simulink library "thermochemical"  (R2017b)
settings: Solver=VariableStepAuto  StartTime=0.0  StopTime=10.0  RelTol=1e-3
values from neighbouring files (symbols this model uses):
  c = conversion_factors()    [blk_clausius_clapeyron.m]    (also in blk_clausius_clapeyron_no_popup.m; blk_cold_room_closed_dry_air.m; blk_reactor_BaCl2_NH3_no_walls.m; blk_reactor_BaCl2_NH3_no_walls_state_space.m)
  cp = metal.cp    [blk_wall_simple.m]    (also in get_metal_properties.m = 390)
  fluid = get_param(blk,'fluid')    [blk_thermodynamic_properties_nonsaturated.m]    (also in blk_thermodynamic_properties_nonsaturated_interpreted.m; blk_thermodynamic_properties_saturated.m; blk_thermodynamic_properties_saturated_interpreted.m; blk_thermodynamic_properties_saturated_mix.m)
  gas = get_material_properties(x.gasName)    [blk_reactor_BaCl2_NH3_cylindrical_no_walls_fun1.m]
  h = get_param(gcb,'ObjectParameters')    [get_param_eval.m]
  rho = metal.rho    [blk_wall_simple.m]    (also in get_metal_properties.m = 8940)
  s = solve(eq,dx,'ReturnConditions',true)    [LMTD_inv.m]    (also in blk_wall_simple.m = get_param_eval(blk,'s'))
  u_gas_at_T_ref = -R * T_ref    [blk_reactor_BaCl2_NH3_no_walls.m]    (also in blk_reactor_BaCl2_NH3_no_walls_state_space.m)
undefined symbols (not defined in the file or in its folder): b_motor, BaCl2, beta, CoolProp, cP_binder, cP_gas, cP_s0, cv, dh_r_0, ENG, heat_exchanger_epsilonNTU_inv_simulink, heat_exchanger_epsilonNTU_simulink, J_motor, K_cin, kappa, Km_motor, La_motor, lookup2D_BreakPoint2, M_binder, N_binder, N_gas_free_volume_init, N_salt, NH3, nh3_v3, nu, P, phase, PID_D_motor, PID_I_motor, PID_P_motor, Ra_motor, Reactor_phase, T, T1, T2, T_init, Tr_init, Tr_ref, U_binder_at_Tr_ref, U_salt_at_X0_Tr_ref, Ur_init, V_void, Valve_regime, Vmax_motor, w_init_motor, X_init
libraries: thermochemical x247, simulink x54, dspsigops x3
(part 5 of 12)

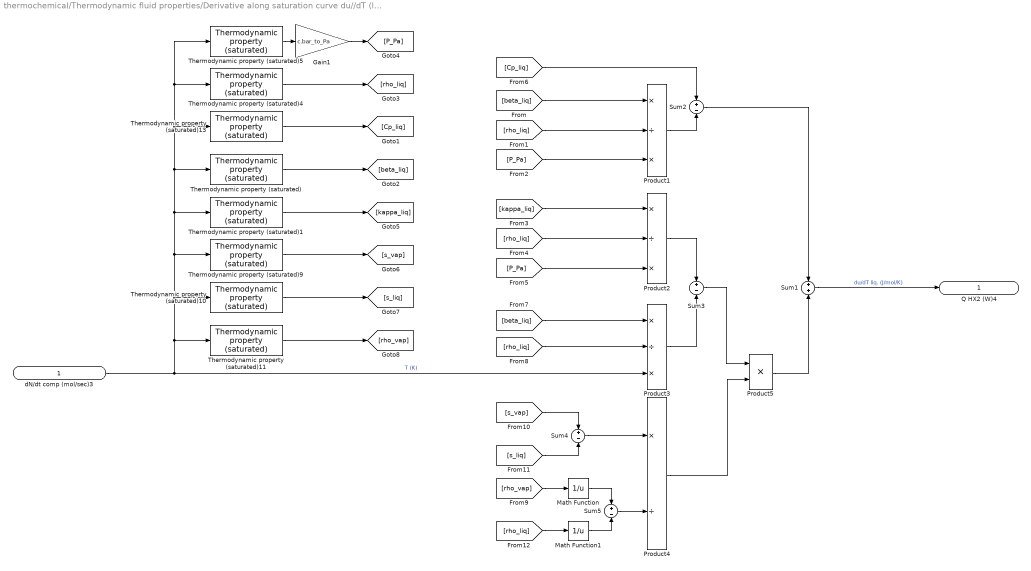
== system thermochemical/Thermodynamic fluid properties/Derivative along saturation curve du//dT (liq.) ==
  dN/dt comp (mol/sec)3 : Inport
  Gain1 : Gain  Gain=c.bar_to_Pa
  Math Function : Math  Operator=reciprocal  SaturateOnIntegerOverflow=on
  Math Function1 : Math  Operator=reciprocal  SaturateOnIntegerOverflow=on
  Product1 : Product  Inputs=*/*
  Product2 : Product  Inputs=*/*
  Product3 : Product  Inputs=*/*
  Product4 : Product  Inputs=*/
  Product5 : Product  Inputs=**
  Sum1 : Sum
  Sum{2..5} (4 alike) : Sum  Inputs=+-
  Thermodynamic property (saturated) : thermochemical/Thermodynamic fluid properties/Thermodynamic  property (saturated)  sel=beta(T) liq. (1/K)  fluid=fluid  lookup1D_BreakPoint1=fluid.sat.T  lookup1D_Data=fluid.sat.liq.beta
      settings: SourceProductName=@ Thermochemical
  Thermodynamic property (saturated)1 : thermochemical/Thermodynamic fluid properties/Thermodynamic  property (saturated)  sel=kappa(T) liq. (1/Pa)  fluid=fluid  lookup1D_BreakPoint1=fluid.sat.T  lookup1D_Data=fluid.sat.liq.kappa
      settings: SourceProductName=@ Thermochemical
  Thermodynamic property (saturated)10 : thermochemical/Thermodynamic fluid properties/Thermodynamic  property (saturated)  sel=s(T) liq. (J/K/mol)  fluid=fluid  lookup1D_BreakPoint1=fluid.sat.T  lookup1D_Data=fluid.sat.liq.s_molar
      settings: SourceProductName=@ Thermochemical
  Thermodynamic property (saturated)11 : thermochemical/Thermodynamic fluid properties/Thermodynamic  property (saturated)  sel=rho(T) vap. (mol/m3)  fluid=fluid  lookup1D_BreakPoint1=fluid.sat.T  lookup1D_Data=fluid.sat.vap.rho_molar
      settings: SourceProductName=@ Thermochemical
  Thermodynamic property (saturated)13 : thermochemical/Thermodynamic fluid properties/Thermodynamic  property (saturated)  sel=Cp(T) liq. (J/K/mol)  fluid=fluid  lookup1D_BreakPoint1=fluid.sat.T  lookup1D_Data=fluid.sat.liq.Cp_molar
      settings: SourceProductName=@ Thermochemical
  Thermodynamic property (saturated)4 : thermochemical/Thermodynamic fluid properties/Thermodynamic  property (saturated)  sel=rho(T) liq. (mol/m3)  fluid=fluid  lookup1D_BreakPoint1=fluid.sat.T  lookup1D_Data=fluid.sat.liq.rho_molar
      settings: SourceProductName=@ Thermochemical
  Thermodynamic property (saturated)5 : thermochemical/Thermodynamic fluid properties/Thermodynamic  property (saturated)  sel=P(T) (bar)  fluid=nh3_v4  lookup1D_BreakPoint1=nh3_v4.sat.T  lookup1D_Data=nh3_v4.sat.Psat
      settings: SourceProductName=@ Thermochemical
  Thermodynamic property (saturated)9 : thermochemical/Thermodynamic fluid properties/Thermodynamic  property (saturated)  sel=s(T) vap. (J/K/mol)  fluid=fluid  lookup1D_BreakPoint1=fluid.sat.T  lookup1D_Data=fluid.sat.vap.s_molar
      settings: SourceProductName=@ Thermochemical
  Q HX2 (W)4 : Outport
  wires:
  Thermodynamic property (saturated)11/1 -> [rho_vap]
  Thermodynamic property (saturated)10/1 -> [s_liq]
  Thermodynamic property (saturated)9/1 -> [s_vap]
  Thermodynamic property (saturated)1/1 -> [kappa_liq]
  Gain1/1 -> [P_Pa]
  Thermodynamic property (saturated)5/1 -> Gain1/1
  Thermodynamic property (saturated)4/1 -> [rho_liq]
  Thermodynamic property (saturated)/1 -> [beta_liq]
  Thermodynamic property (saturated)13/1 -> [Cp_liq]
  Sum1/1 -> Q HX2 (W)4/1  "du/dT liq. (J/mol/K)"
  [Cp_liq] -> Sum2/1
  Product1/1 -> Sum2/2
  [beta_liq] -> Product1/1
  [rho_liq] -> Product1/2
  Sum2/1 -> Sum1/1
  [P_Pa] -> Product1/3
  dN/dt comp (mol/sec)3/1 -> Product3/3, Thermodynamic property (saturated)5/1, Thermodynamic property (saturated)4/1, Thermodynamic property (saturated)13/1, Thermodynamic property (saturated)/1, Thermodynamic property (saturated)1/1, Thermodynamic property (saturated)9/1, Thermodynamic property (saturated)10/1, Thermodynamic property (saturated)11/1  "T (K)"
  [kappa_liq] -> Product2/1
  [rho_liq] -> Product2/2
  [P_Pa] -> Product2/3
  Product2/1 -> Sum3/1
  [rho_liq] -> Product3/2
  [beta_liq] -> Product3/1
  Product3/1 -> Sum3/2
  [s_vap] -> Sum4/1
  [s_liq] -> Sum4/2
  Sum4/1 -> Product4/1
  Sum5/1 -> Product4/2
  [rho_liq] -> Math Function1/1
  [rho_vap] -> Math Function/1
  Math Function/1 -> Sum5/1
  Math Function1/1 -> Sum5/2
  Sum3/1 -> Product5/1
  Product4/1 -> Product5/2
  Product5/1 -> Sum1/2

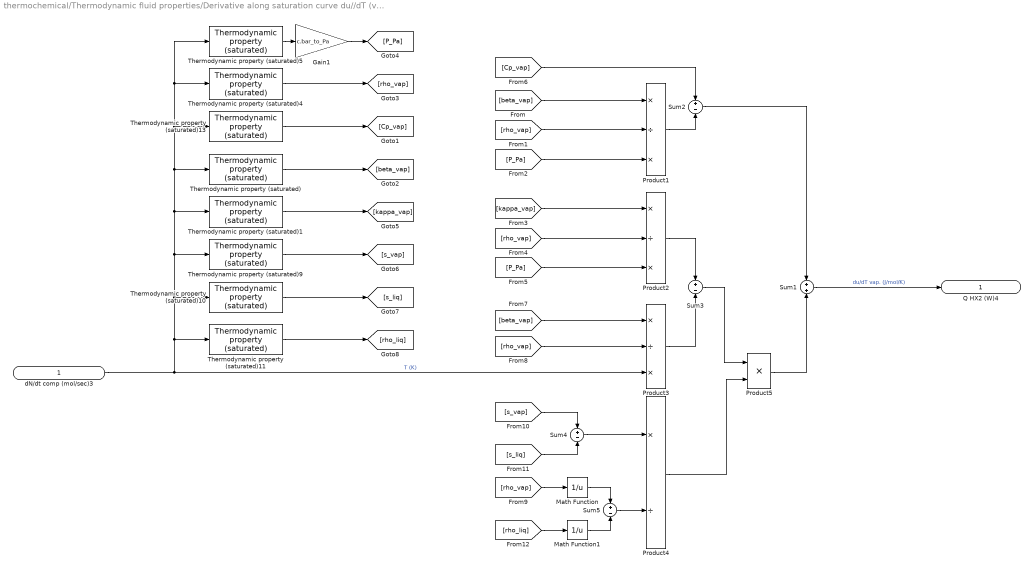
== system thermochemical/Thermodynamic fluid properties/Derivative along saturation curve du//dT (vap.) ==
  dN/dt comp (mol/sec)3 : Inport
  Gain1 : Gain  Gain=c.bar_to_Pa
  Math Function : Math  Operator=reciprocal  SaturateOnIntegerOverflow=on
  Math Function1 : Math  Operator=reciprocal  SaturateOnIntegerOverflow=on
  Product1 : Product  Inputs=*/*
  Product2 : Product  Inputs=*/*
  Product3 : Product  Inputs=*/*
  Product4 : Product  Inputs=*/
  Product5 : Product  Inputs=**
  Sum1 : Sum
  Sum{2..5} (4 alike) : Sum  Inputs=+-
  Thermodynamic property (saturated) : thermochemical/Thermodynamic fluid properties/Thermodynamic  property (saturated)  sel=beta(T) vap. (1/K)  fluid=fluid  lookup1D_BreakPoint1=fluid.sat.T  lookup1D_Data=fluid.sat.vap.beta
      settings: SourceProductName=@ Thermochemical
  Thermodynamic property (saturated)1 : thermochemical/Thermodynamic fluid properties/Thermodynamic  property (saturated)  sel=kappa(T) vap. (1/Pa)  fluid=fluid  lookup1D_BreakPoint1=fluid.sat.T  lookup1D_Data=fluid.sat.vap.kappa
      settings: SourceProductName=@ Thermochemical
  Thermodynamic property (saturated)10 : thermochemical/Thermodynamic fluid properties/Thermodynamic  property (saturated)  sel=s(T) liq. (J/K/mol)  fluid=fluid  lookup1D_BreakPoint1=fluid.sat.T  lookup1D_Data=fluid.sat.liq.s_molar
      settings: SourceProductName=@ Thermochemical
  Thermodynamic property (saturated)11 : thermochemical/Thermodynamic fluid properties/Thermodynamic  property (saturated)  sel=rho(T) liq. (mol/m3)  fluid=fluid  lookup1D_BreakPoint1=fluid.sat.T  lookup1D_Data=fluid.sat.liq.rho_molar
      settings: SourceProductName=@ Thermochemical
  Thermodynamic property (saturated)13 : thermochemical/Thermodynamic fluid properties/Thermodynamic  property (saturated)  sel=Cp(T) vap. (J/K/mol)  fluid=fluid  lookup1D_BreakPoint1=fluid.sat.T  lookup1D_Data=fluid.sat.vap.Cp_molar
      settings: SourceProductName=@ Thermochemical
  Thermodynamic property (saturated)4 : thermochemical/Thermodynamic fluid properties/Thermodynamic  property (saturated)  sel=rho(T) vap. (mol/m3)  fluid=fluid  lookup1D_BreakPoint1=fluid.sat.T  lookup1D_Data=fluid.sat.vap.rho_molar
      settings: SourceProductName=@ Thermochemical
  Thermodynamic property (saturated)5 : thermochemical/Thermodynamic fluid properties/Thermodynamic  property (saturated)  sel=P(T) (bar)  fluid=nh3_v4  lookup1D_BreakPoint1=nh3_v4.sat.T  lookup1D_Data=nh3_v4.sat.Psat
      settings: SourceProductName=@ Thermochemical
  Thermodynamic property (saturated)9 : thermochemical/Thermodynamic fluid properties/Thermodynamic  property (saturated)  sel=s(T) vap. (J/K/mol)  fluid=fluid  lookup1D_BreakPoint1=fluid.sat.T  lookup1D_Data=fluid.sat.vap.s_molar
      settings: SourceProductName=@ Thermochemical
  Q HX2 (W)4 : Outport
  wires:
  Product5/1 -> Sum1/2
  Product4/1 -> Product5/2
  Sum3/1 -> Product5/1
  Math Function1/1 -> Sum5/2
  Math Function/1 -> Sum5/1
  [rho_vap] -> Math Function/1
  [rho_liq] -> Math Function1/1
  Sum5/1 -> Product4/2
  Sum4/1 -> Product4/1
  [s_liq] -> Sum4/2
  [s_vap] -> Sum4/1
  Product3/1 -> Sum3/2
  [beta_vap] -> Product3/1
  [rho_vap] -> Product3/2
  Product2/1 -> Sum3/1
  [P_Pa] -> Product2/3
  [rho_vap] -> Product2/2
  [kappa_vap] -> Product2/1
  dN/dt comp (mol/sec)3/1 -> Thermodynamic property (saturated)11/1, Thermodynamic property (saturated)10/1, Thermodynamic property (saturated)9/1, Thermodynamic property (saturated)1/1, Thermodynamic property (saturated)/1, Thermodynamic property (saturated)13/1, Thermodynamic property (saturated)4/1, Thermodynamic property (saturated)5/1, Product3/3  "T (K)"
  [P_Pa] -> Product1/3
  Sum2/1 -> Sum1/1
  [rho_vap] -> Product1/2
  [beta_vap] -> Product1/1
  Product1/1 -> Sum2/2
  [Cp_vap] -> Sum2/1
  Sum1/1 -> Q HX2 (W)4/1  "du/dT vap. (J/mol/K)"
  Thermodynamic property (saturated)13/1 -> [Cp_vap]
  Thermodynamic property (saturated)/1 -> [beta_vap]
  Thermodynamic property (saturated)4/1 -> [rho_vap]
  Thermodynamic property (saturated)5/1 -> Gain1/1
  Gain1/1 -> [P_Pa]
  Thermodynamic property (saturated)1/1 -> [kappa_vap]
  Thermodynamic property (saturated)9/1 -> [s_vap]
  Thermodynamic property (saturated)10/1 -> [s_liq]
  Thermodynamic property (saturated)11/1 -> [rho_liq]

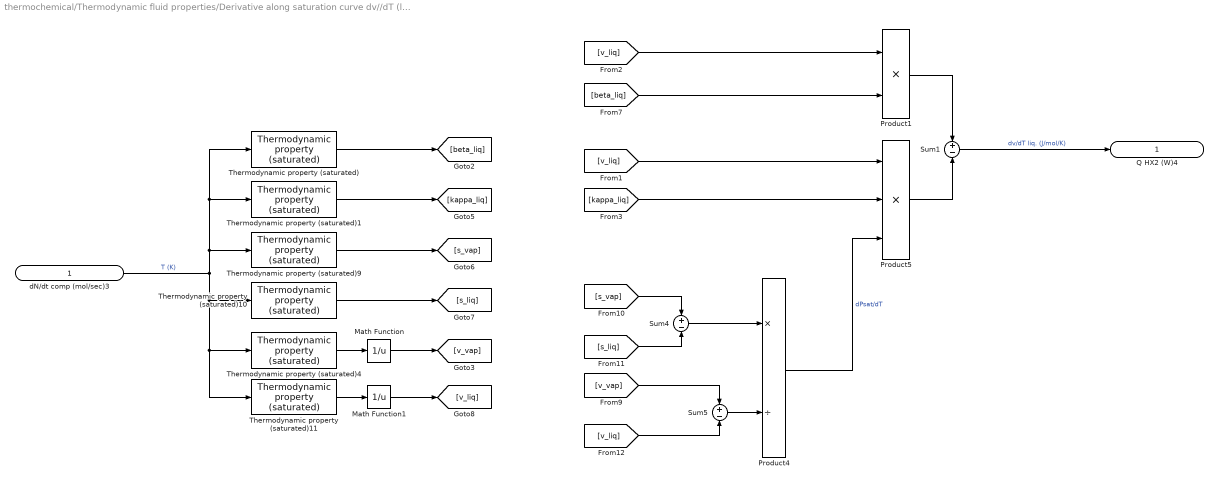
== system thermochemical/Thermodynamic fluid properties/Derivative along saturation curve dv//dT (liq.) ==
  dN/dt comp (mol/sec)3 : Inport
  Math Function : Math  Operator=reciprocal  SaturateOnIntegerOverflow=on
  Math Function1 : Math  Operator=reciprocal  SaturateOnIntegerOverflow=on
  Product1 : Product  Inputs=**
  Product4 : Product  Inputs=*/
  Product5 : Product  Inputs=***
  Sum1 : Sum  Inputs=+-
  Sum4 : Sum  Inputs=+-
  Sum5 : Sum  Inputs=+-
  Thermodynamic property (saturated) : thermochemical/Thermodynamic fluid properties/Thermodynamic  property (saturated)  sel=beta(T) liq. (1/K)  fluid=fluid  lookup1D_BreakPoint1=fluid.sat.T  lookup1D_Data=fluid.sat.liq.beta
      settings: SourceProductName=@ Thermochemical
  Thermodynamic property (saturated)1 : thermochemical/Thermodynamic fluid properties/Thermodynamic  property (saturated)  sel=kappa(T) liq. (1/Pa)  fluid=fluid  lookup1D_BreakPoint1=fluid.sat.T  lookup1D_Data=fluid.sat.liq.kappa
      settings: SourceProductName=@ Thermochemical
  Thermodynamic property (saturated)10 : thermochemical/Thermodynamic fluid properties/Thermodynamic  property (saturated)  sel=s(T) liq. (J/K/mol)  fluid=fluid  lookup1D_BreakPoint1=fluid.sat.T  lookup1D_Data=fluid.sat.liq.s_molar
      settings: SourceProductName=@ Thermochemical
  Thermodynamic property (saturated)11 : thermochemical/Thermodynamic fluid properties/Thermodynamic  property (saturated)  sel=rho(T) liq. (mol/m3)  fluid=fluid  lookup1D_BreakPoint1=fluid.sat.T  lookup1D_Data=fluid.sat.liq.rho_molar
      settings: SourceProductName=@ Thermochemical
  Thermodynamic property (saturated)4 : thermochemical/Thermodynamic fluid properties/Thermodynamic  property (saturated)  sel=rho(T) vap. (mol/m3)  fluid=fluid  lookup1D_BreakPoint1=fluid.sat.T  lookup1D_Data=fluid.sat.vap.rho_molar
      settings: SourceProductName=@ Thermochemical
  Thermodynamic property (saturated)9 : thermochemical/Thermodynamic fluid properties/Thermodynamic  property (saturated)  sel=s(T) vap. (J/K/mol)  fluid=fluid  lookup1D_BreakPoint1=fluid.sat.T  lookup1D_Data=fluid.sat.vap.s_molar
      settings: SourceProductName=@ Thermochemical
  Q HX2 (W)4 : Outport
  wires:
  Product1/1 -> Sum1/1
  [v_liq] -> Product1/1
  [v_liq] -> Product5/1
  Math Function1/1 -> [v_liq]
  Math Function/1 -> [v_vap]
  Product5/1 -> Sum1/2
  Product4/1 -> Product5/3  "dPsat/dT"
  [v_liq] -> Sum5/2
  [v_vap] -> Sum5/1
  Sum5/1 -> Product4/2
  Sum4/1 -> Product4/1
  [s_liq] -> Sum4/2
  [s_vap] -> Sum4/1
  [beta_liq] -> Product1/2
  [kappa_liq] -> Product5/2
  dN/dt comp (mol/sec)3/1 -> Thermodynamic property (saturated)9/1, Thermodynamic property (saturated)1/1, Thermodynamic property (saturated)/1, Thermodynamic property (saturated)10/1, Thermodynamic property (saturated)4/1, Thermodynamic property (saturated)11/1  "T (K)"
  Sum1/1 -> Q HX2 (W)4/1  "dv/dT liq. (J/mol/K)"
  Thermodynamic property (saturated)/1 -> [beta_liq]
  Thermodynamic property (saturated)4/1 -> Math Function/1
  Thermodynamic property (saturated)1/1 -> [kappa_liq]
  Thermodynamic property (saturated)9/1 -> [s_vap]
  Thermodynamic property (saturated)10/1 -> [s_liq]
  Thermodynamic property (saturated)11/1 -> Math Function1/1

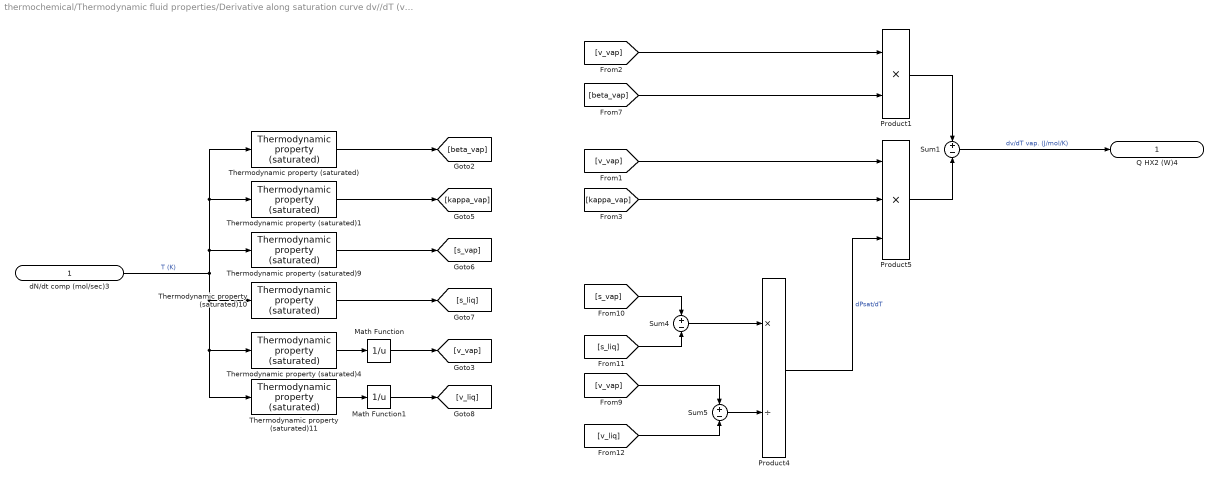
== system thermochemical/Thermodynamic fluid properties/Derivative along saturation curve dv//dT (vap.) ==
  dN/dt comp (mol/sec)3 : Inport
  Math Function : Math  Operator=reciprocal  SaturateOnIntegerOverflow=on
  Math Function1 : Math  Operator=reciprocal  SaturateOnIntegerOverflow=on
  Product1 : Product  Inputs=**
  Product4 : Product  Inputs=*/
  Product5 : Product  Inputs=***
  Sum1 : Sum  Inputs=+-
  Sum4 : Sum  Inputs=+-
  Sum5 : Sum  Inputs=+-
  Thermodynamic property (saturated) : thermochemical/Thermodynamic fluid properties/Thermodynamic  property (saturated)  sel=beta(T) vap. (1/K)  fluid=fluid  lookup1D_BreakPoint1=fluid.sat.T  lookup1D_Data=fluid.sat.vap.beta
      settings: SourceProductName=@ Thermochemical
  Thermodynamic property (saturated)1 : thermochemical/Thermodynamic fluid properties/Thermodynamic  property (saturated)  sel=kappa(T) vap. (1/Pa)  fluid=fluid  lookup1D_BreakPoint1=fluid.sat.T  lookup1D_Data=fluid.sat.vap.kappa
      settings: SourceProductName=@ Thermochemical
  Thermodynamic property (saturated)10 : thermochemical/Thermodynamic fluid properties/Thermodynamic  property (saturated)  sel=s(T) liq. (J/K/mol)  fluid=fluid  lookup1D_BreakPoint1=fluid.sat.T  lookup1D_Data=fluid.sat.liq.s_molar
      settings: SourceProductName=@ Thermochemical
  Thermodynamic property (saturated)11 : thermochemical/Thermodynamic fluid properties/Thermodynamic  property (saturated)  sel=rho(T) liq. (mol/m3)  fluid=fluid  lookup1D_BreakPoint1=fluid.sat.T  lookup1D_Data=fluid.sat.liq.rho_molar
      settings: SourceProductName=@ Thermochemical
  Thermodynamic property (saturated)4 : thermochemical/Thermodynamic fluid properties/Thermodynamic  property (saturated)  sel=rho(T) vap. (mol/m3)  fluid=fluid  lookup1D_BreakPoint1=fluid.sat.T  lookup1D_Data=fluid.sat.vap.rho_molar
      settings: SourceProductName=@ Thermochemical
  Thermodynamic property (saturated)9 : thermochemical/Thermodynamic fluid properties/Thermodynamic  property (saturated)  sel=s(T) vap. (J/K/mol)  fluid=fluid  lookup1D_BreakPoint1=fluid.sat.T  lookup1D_Data=fluid.sat.vap.s_molar
      settings: SourceProductName=@ Thermochemical
  Q HX2 (W)4 : Outport
  wires:
  Thermodynamic property (saturated)11/1 -> Math Function1/1
  Thermodynamic property (saturated)10/1 -> [s_liq]
  Thermodynamic property (saturated)9/1 -> [s_vap]
  Thermodynamic property (saturated)1/1 -> [kappa_vap]
  Thermodynamic property (saturated)4/1 -> Math Function/1
  Thermodynamic property (saturated)/1 -> [beta_vap]
  Sum1/1 -> Q HX2 (W)4/1  "dv/dT vap. (J/mol/K)"
  dN/dt comp (mol/sec)3/1 -> Thermodynamic property (saturated)11/1, Thermodynamic property (saturated)4/1, Thermodynamic property (saturated)10/1, Thermodynamic property (saturated)/1, Thermodynamic property (saturated)1/1, Thermodynamic property (saturated)9/1  "T (K)"
  [kappa_vap] -> Product5/2
  [beta_vap] -> Product1/2
  [s_vap] -> Sum4/1
  [s_liq] -> Sum4/2
  Sum4/1 -> Product4/1
  Sum5/1 -> Product4/2
  [v_vap] -> Sum5/1
  [v_liq] -> Sum5/2
  Product4/1 -> Product5/3  "dPsat/dT"
  Product5/1 -> Sum1/2
  Math Function/1 -> [v_vap]
  Math Function1/1 -> [v_liq]
  [v_vap] -> Product5/1
  [v_vap] -> Product1/1
  Product1/1 -> Sum1/1

== system thermochemical/Thermodynamic fluid properties/Derivative in the two-phase region ∂u//∂T|v ==
  dN/dt comp (mol/sec)1 : Inport
  dN/dt comp (mol/sec)2 : Inport  Port=2
  Derivative along saturation curve du/dT (liq.) : thermochemical/Thermodynamic fluid properties/Derivative along saturation curve du//dT (liq.)  fluid=fluid
      settings: SourceProductName=@ Thermochemical
  Derivative along saturation curve du/dT (vap.) : thermochemical/Thermodynamic fluid properties/Derivative along saturation curve du//dT (vap.)  fluid=fluid
      settings: SourceProductName=@ Thermochemical
  Derivative in the two-phase region ∂χ/∂T|v : thermochemical/Thermodynamic fluid properties/Derivative in the two-phase region ∂χ//∂T|v  fluid=fluid
      settings: SourceProductName=@ Thermochemical
  Product1 : Product  Inputs=**
  Product2 : Product  Inputs=**
  Sum1 : Sum  Inputs=+-
  Sum2 : Sum  Inputs=+-
  Sum3 : Sum  Inputs=+++
  Thermodynamic property (saturated) : thermochemical/Thermodynamic fluid properties/Thermodynamic  property (saturated)  sel=u(T) vap. (J/mol)  fluid=fluid  lookup1D_BreakPoint1=fluid.sat.T  lookup1D_Data=fluid.sat.vap.u_molar
      settings: SourceProductName=@ Thermochemical
  Thermodynamic property (saturated)1 : thermochemical/Thermodynamic fluid properties/Thermodynamic  property (saturated)  sel=u(T) liq. (J/mol)  fluid=nh3_v4  lookup1D_BreakPoint1=nh3_v4.sat.T  lookup1D_Data=nh3_v4.sat.liq.u_molar
      settings: SourceProductName=@ Thermochemical
  Q HX2 (W)4 : Outport
  wires:
  Sum3/1 -> Q HX2 (W)4/1  "∂u/∂T|v (J/mol/K) (two-phase)"
  dN/dt comp (mol/sec)2/1 -> Derivative in the two-phase region ∂χ/∂T|v/2, Product2/1  "χ (0..1)"
  Derivative along saturation curve du/dT (vap.)/1 -> Sum1/1
  Derivative along saturation curve du/dT (liq.)/1 -> Sum3/2, Sum1/2  "∂u(liq)/∂T|v"
  Sum1/1 -> Product2/2  "∂u(vap)/∂T|v - ∂u(liq)/∂T|v"
  dN/dt comp (mol/sec)1/1 -> Thermodynamic property (saturated)/1, Thermodynamic property (saturated)1/1, Derivative in the two-phase region ∂χ/∂T|v/1, Derivative along saturation curve du/dT (liq.)/1, Derivative along saturation curve du/dT (vap.)/1  "T (K)"
  Product2/1 -> Sum3/1  "χ*[∂u(vap)/∂T|v - ∂u(liq)/∂T|v]"
  Derivative in the two-phase region ∂χ/∂T|v/1 -> Product1/2  "∂χ/∂T|v (1/K)"
  Thermodynamic property (saturated)1/1 -> Sum2/2
  Thermodynamic property (saturated)/1 -> Sum2/1
  Sum2/1 -> Product1/1  "u(vap) - u(liq)"
  Product1/1 -> Sum3/3  "∂χ/∂T|v * [u(vap) - u(liq)]"

== system thermochemical/Thermodynamic fluid properties/Derivative in the two-phase region ∂u//∂v|T ==
  dN/dt comp (mol/sec)3 : Inport
  Derivative in the two-phase region ∂χ/∂v|T : thermochemical/Thermodynamic fluid properties/Derivative in the two-phase region ∂χ//∂v|T  fluid=fluid
      settings: SourceProductName=@ Thermochemical
  Product : Product  Inputs=**
  Sum1 : Sum  Inputs=+-
  Thermodynamic property (saturated) : thermochemical/Thermodynamic fluid properties/Thermodynamic  property (saturated)  sel=u(T) vap. (J/mol)  fluid=fluid  lookup1D_BreakPoint1=fluid.sat.T  lookup1D_Data=fluid.sat.vap.u_molar
      settings: SourceProductName=@ Thermochemical
  Thermodynamic property (saturated)1 : thermochemical/Thermodynamic fluid properties/Thermodynamic  property (saturated)  sel=u(T) liq. (J/mol)  fluid=nh3_v4  lookup1D_BreakPoint1=nh3_v4.sat.T  lookup1D_Data=nh3_v4.sat.liq.u_molar
      settings: SourceProductName=@ Thermochemical
  Q HX2 (W)4 : Outport
  wires:
  Thermodynamic property (saturated)1/1 -> Sum1/2
  Product/1 -> Q HX2 (W)4/1  "∂u/∂v|T (J/m³) (two-phase)"
  Thermodynamic property (saturated)/1 -> Sum1/1
  Sum1/1 -> Product/1
  dN/dt comp (mol/sec)3/1 -> Derivative in the two-phase region ∂χ/∂v|T/1, Thermodynamic property (saturated)1/1, Thermodynamic property (saturated)/1  "T (K)"
  Derivative in the two-phase region ∂χ/∂v|T/1 -> Product/2

== system thermochemical/Thermodynamic fluid properties/Derivative in the two-phase region ∂χ//∂T|v ==
  dN/dt comp (mol/sec)3 : Inport
  dN/dt comp (mol/sec)1 : Inport  Port=2
  Derivative along saturation curve dv/dT (liq.) : thermochemical/Thermodynamic fluid properties/Derivative along saturation curve dv//dT (liq.)  fluid=fluid
      settings: SourceProductName=@ Thermochemical
  Derivative along saturation curve dv/dT (vap.) : thermochemical/Thermodynamic fluid properties/Derivative along saturation curve dv//dT (vap.)  fluid=fluid
      settings: SourceProductName=@ Thermochemical
  Math Function : Math  Operator=reciprocal  SaturateOnIntegerOverflow=on
  Math Function1 : Math  Operator=reciprocal  SaturateOnIntegerOverflow=on
  Product1 : Product  Inputs=*/
  Product2 : Product  Inputs=**
  Sum1 : Sum  Inputs=+-
  Sum2 : Sum  Inputs=+-
  Sum3 : Sum
  Thermodynamic property (saturated)2 : thermochemical/Thermodynamic fluid properties/Thermodynamic  property (saturated)  sel=rho(T) vap. (mol/m3)  fluid=fluid  lookup1D_BreakPoint1=fluid.sat.T  lookup1D_Data=fluid.sat.vap.rho_molar
      settings: SourceProductName=@ Thermochemical
  Thermodynamic property (saturated)3 : thermochemical/Thermodynamic fluid properties/Thermodynamic  property (saturated)  sel=rho(T) liq. (mol/m3)  fluid=nh3_v4  lookup1D_BreakPoint1=nh3_v4.sat.T  lookup1D_Data=nh3_v4.sat.liq.rho_molar
      settings: SourceProductName=@ Thermochemical
  Q HX2 (W)4 : Outport
  wires:
  Product1/1 -> Q HX2 (W)4/1  "∂χ/∂T|v (1/K) (two-phase)"
  Thermodynamic property (saturated)3/1 -> Math Function/1
  dN/dt comp (mol/sec)3/1 -> Thermodynamic property (saturated)2/1, Thermodynamic property (saturated)3/1, Derivative along saturation curve dv/dT (liq.)/1, Derivative along saturation curve dv/dT (vap.)/1  "T (K)"
  Thermodynamic property (saturated)2/1 -> Math Function1/1
  Sum2/1 -> Product1/2
  Math Function/1 -> Sum2/1
  Math Function1/1 -> Sum2/2
  dN/dt comp (mol/sec)1/1 -> Product2/1  "χ (0..1)"
  Derivative along saturation curve dv/dT (vap.)/1 -> Sum1/1
  Derivative along saturation curve dv/dT (liq.)/1 -> Sum3/2, Sum1/2
  Sum1/1 -> Product2/2
  Product2/1 -> Sum3/1
  Sum3/1 -> Product1/1

== system thermochemical/Thermodynamic fluid properties/Derivative in the two-phase region ∂χ//∂v|T ==
  dN/dt comp (mol/sec)3 : Inport
  Math Function : Math  Operator=reciprocal  SaturateOnIntegerOverflow=on
  Math Function1 : Math  Operator=reciprocal  SaturateOnIntegerOverflow=on
  Math Function2 : Math  Operator=reciprocal  SaturateOnIntegerOverflow=on
  Sum2 : Sum  Inputs=+-
  Thermodynamic property (saturated)2 : thermochemical/Thermodynamic fluid properties/Thermodynamic  property (saturated)  sel=rho(T) vap. (mol/m3)  fluid=fluid  lookup1D_BreakPoint1=fluid.sat.T  lookup1D_Data=fluid.sat.vap.rho_molar
      settings: SourceProductName=@ Thermochemical
  Thermodynamic property (saturated)3 : thermochemical/Thermodynamic fluid properties/Thermodynamic  property (saturated)  sel=rho(T) liq. (mol/m3)  fluid=nh3_v4  lookup1D_BreakPoint1=nh3_v4.sat.T  lookup1D_Data=nh3_v4.sat.liq.rho_molar
      settings: SourceProductName=@ Thermochemical
  Q HX2 (W)4 : Outport
  wires:
  Math Function1/1 -> Sum2/2
  Math Function/1 -> Sum2/1
  Sum2/1 -> Math Function2/1
  Thermodynamic property (saturated)3/1 -> Math Function1/1
  dN/dt comp (mol/sec)3/1 -> Thermodynamic property (saturated)2/1, Thermodynamic property (saturated)3/1  "T (K)"
  Thermodynamic property (saturated)2/1 -> Math Function/1
  Math Function2/1 -> Q HX2 (W)4/1  "∂χ/∂v|T (mol/m³) (two-phase)"

== system thermochemical/Thermodynamic fluid properties/Enthalpy of ideal gas ==
  In2 : Inport
  3 : Constant  Value=T_ref
  Cp : Gain  Gain=cP_gas
  Enthalpy at reference temperautre T_ref : Constant  Value=h_gas_at_T_ref
  Sum5 : Sum  Inputs=|+-
  Sum6 : Sum  Inputs=|++
  Out2 : Outport
  wires:
  Enthalpy at reference temperautre T_ref/1 -> Sum6/2
  Cp/1 -> Sum6/1
  Sum6/1 -> Out2/1  "h gas (ideal) (J/mol)"
  In2/1 -> Sum5/1  "T (K)"
  3/1 -> Sum5/2
  Sum5/1 -> Cp/1

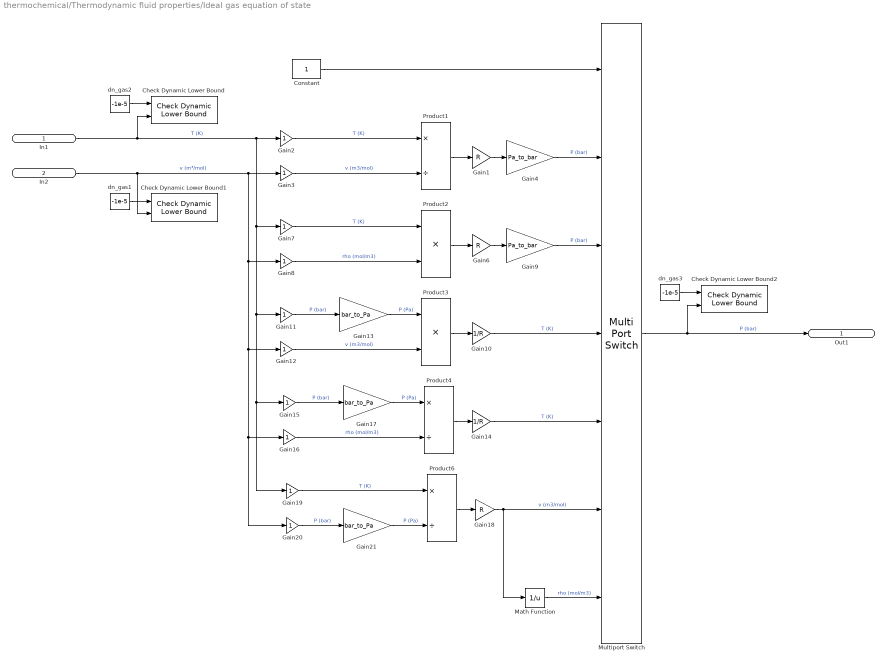
== system thermochemical/Thermodynamic fluid properties/Ideal gas equation of state ==
  In1 : Inport
  In2 : Inport  Port=2
  Check Dynamic Lower Bound : simulink/Model Verification/Check Dynamic  Lower Bound  Description=min < u  Enabled=on  stopWhenAssertionFail=on  export=off  icon=graphic
      settings: SourceProductName=Simulink  SourceProductBaseCode=SL
  Check Dynamic Lower Bound1 : simulink/Model Verification/Check Dynamic  Lower Bound  Description=min < u  Enabled=on  stopWhenAssertionFail=on  export=off  icon=graphic
      settings: SourceProductName=Simulink  SourceProductBaseCode=SL
  Check Dynamic Lower Bound2 : simulink/Model Verification/Check Dynamic  Lower Bound  Description=min < u  Enabled=on  stopWhenAssertionFail=on  export=off  icon=graphic
      settings: SourceProductName=Simulink  SourceProductBaseCode=SL
  Constant : Constant
  Gain1 : Gain  Gain=R
  Gain10 : Gain  Gain=1/R
  Gain{2..3,7..8,11..12,15..16,19..20} (10 alike) : Gain
  Gain13 : Gain  Gain=bar_to_Pa
  Gain14 : Gain  Gain=1/R
  Gain17 : Gain  Gain=bar_to_Pa
  Gain18 : Gain  Gain=R
  Gain21 : Gain  Gain=bar_to_Pa
  Gain4 : Gain  Gain=Pa_to_bar
  Gain6 : Gain  Gain=R
  Gain9 : Gain  Gain=Pa_to_bar
  Math Function : Math  Operator=reciprocal  SaturateOnIntegerOverflow=on
  Multiport Switch : MultiPortSwitch  Inputs=6
  Product1 : Product  Inputs=*/
  Product2 : Product  Inputs=**
  Product3 : Product  Inputs=**
  Product4 : Product  Inputs=*/
  Product6 : Product  Inputs=*/
  dn_gas1 : Constant  Value=-1e-5
  dn_gas2 : Constant  Value=-1e-5
  dn_gas3 : Constant  Value=-1e-5
  Out1 : Outport
  wires:
  dn_gas2/1 -> Check Dynamic Lower Bound/1
  Constant/1 -> Multiport Switch/1
  Product1/1 -> Gain1/1
  Gain2/1 -> Product1/1  "T (K)"
  Gain3/1 -> Product1/2  "v (m3/mol)"
  Gain1/1 -> Gain4/1
  Gain4/1 -> Multiport Switch/2  "P (bar)"
  Gain9/1 -> Multiport Switch/3  "P (bar)"
  Gain6/1 -> Gain9/1
  Gain8/1 -> Product2/2  "rho (mol/m3)"
  Gain7/1 -> Product2/1  "T (K)"
  Product2/1 -> Gain6/1
  Product3/1 -> Gain10/1
  Gain11/1 -> Gain13/1  "P (bar)"
  Gain12/1 -> Product3/2  "v (m3/mol)"
  Gain10/1 -> Multiport Switch/4  "T (K)"
  Gain13/1 -> Product3/1  "P (Pa)"
  Gain17/1 -> Product4/1  "P (Pa)"
  Gain14/1 -> Multiport Switch/5  "T (K)"
  Gain16/1 -> Product4/2  "rho (mol/m3)"
  Gain15/1 -> Gain17/1  "P (bar)"
  Product4/1 -> Gain14/1
  Product6/1 -> Gain18/1
  Gain19/1 -> Product6/1  "T (K)"
  Gain20/1 -> Gain21/1  "P (bar)"
  Gain18/1 -> Multiport Switch/6, Math Function/1  "v (m3/mol)"
  Gain21/1 -> Product6/2  "P (Pa)"
  In1/1 -> Check Dynamic Lower Bound/2, Gain7/1, Gain19/1, Gain15/1, Gain11/1, Gain2/1  "T (K)"
  Math Function/1 -> Multiport Switch/7  "rho (mol/m3)"
  In2/1 -> Check Dynamic Lower Bound1/2, Gain8/1, Gain12/1, Gain20/1, Gain16/1, Gain3/1  "v (m³/mol)"
  dn_gas1/1 -> Check Dynamic Lower Bound1/1
  dn_gas3/1 -> Check Dynamic Lower Bound2/1
  Multiport Switch/1 -> Check Dynamic Lower Bound2/2, Out1/1  "P (bar)"

== system thermochemical/Thermodynamic fluid properties/Internal energy of ideal gas ==
  In2 : Inport
  3 : Constant  Value=T_ref
  Cv : Gain  Gain=Cv_gas
  Internal energy at reference temperautre T_ref : Constant  Value=u_gas_at_T_ref
  Sum5 : Sum  Inputs=|+-
  Sum6 : Sum  Inputs=|++
  Out2 : Outport
  wires:
  Sum5/1 -> Cv/1
  3/1 -> Sum5/2
  In2/1 -> Sum5/1  "T (K)"
  Sum6/1 -> Out2/1  "u gas (ideal) (J/mol)"
  Cv/1 -> Sum6/1
  Internal energy at reference temperautre T_ref/1 -> Sum6/2

== system thermochemical/Thermodynamic fluid properties/Thermodynamic property (non-saturated) ==
  In1 : Inport
  In2 : Inport  Port=2
  Subsystem1 : Subsystem
  Out1 : Outport
  wires:
  Subsystem1/1(Out1) -> Out1/1  "v (m³/mol)"
  In1/1 -> Subsystem1/1(In1)  "T (K)"
  In2/1 -> Subsystem1/2(In2)  "P (bar)"

== system thermochemical/Thermodynamic fluid properties/Thermodynamic property (non-saturated) (it uses CoolProp library) ==
  In1 : Inport
  In2 : Inport  Port=2
  Subsystem1 : Subsystem
  Out1 : Outport
  wires:
  In2/1 -> Subsystem1/2(In2)  "P (bar)"
  In1/1 -> Subsystem1/1(In1)  "T (K)"
  Subsystem1/1(Out1) -> Out1/1  "v (m³/mol)"

== system thermochemical/Thermodynamic fluid properties/Thermodynamic property (saturated) ==
  In1 : Inport
  Subsystem1 : Subsystem
  Out1 : Outport
  wires:
  In1/1 -> Subsystem1/1(In1)  "T (K)"
  Subsystem1/1(Out1) -> Out1/1  "P(T) (bar)"

== system thermochemical/Thermodynamic fluid properties/Thermodynamic property (saturated) (it uses CoolProp library) ==
  In1 : Inport
  Subsystem1 : Subsystem
  Out1 : Outport
  wires:
  In1/1 -> Subsystem1/1(In1)  "T (K)"
  Subsystem1/1(Out1) -> Out1/1  "P(T) (bar)"

== system thermochemical/Thermodynamic fluid properties/Thermodynamic property (saturated vapor-liquid mix) ==
  In1 : Inport
  In2 : Inport  Port=2
  Check Dynamic Range : simulink/Model Verification/Check  Dynamic Range  Description=min < u < max  enabled=on  stopWhenAssertionFail=off  export=off  icon=graphic
      settings: SourceProductName=Simulink  SourceProductBaseCode=SL
  Subsystem1 : Subsystem
  dn_gas2 : Constant  Value=1+eps
  dn_gas3 : Constant  Value=-eps
  Out1 : Outport
  wires:
  In1/1 -> Subsystem1/1(T(K))  "T(K)"
  In2/1 -> Subsystem1/2(vapor quality (0..1)), Check Dynamic Range/3  "vapor quality (0..1)"
  Subsystem1/1(Out1) -> Out1/1  "h(T) mix (J/mol)"
  dn_gas2/1 -> Check Dynamic Range/1
  dn_gas3/1 -> Check Dynamic Range/2

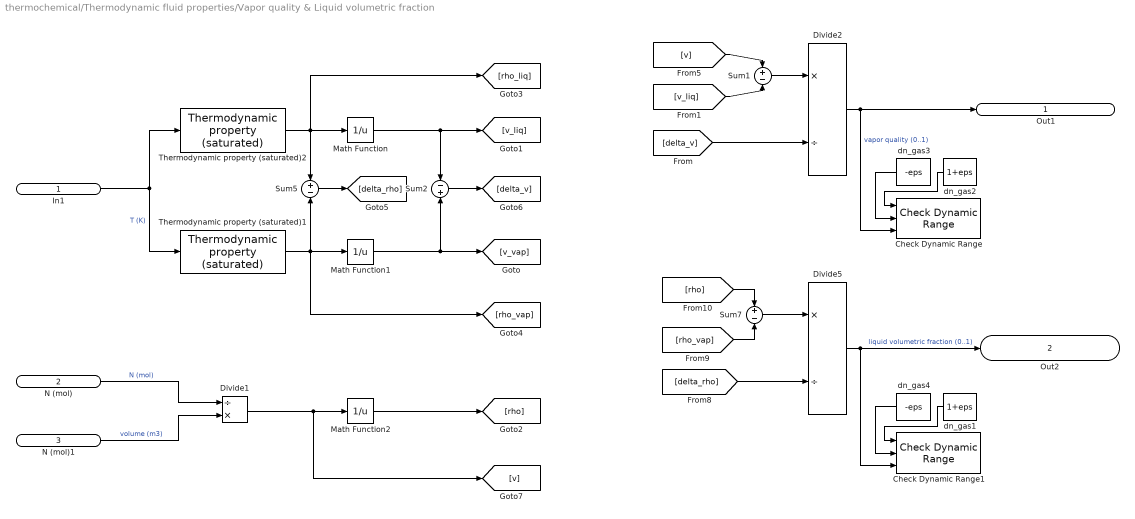
== system thermochemical/Thermodynamic fluid properties/Vapor quality & Liquid volumetric fraction ==
  In1 : Inport
  N (mol) : Inport  Port=2
  N (mol)1 : Inport  Port=3
  Check Dynamic Range : simulink/Model Verification/Check  Dynamic Range  Description=min < u < max  enabled=on  stopWhenAssertionFail=on  export=off  icon=graphic
      settings: SourceProductName=Simulink  SourceProductBaseCode=SL
  Check Dynamic Range1 : simulink/Model Verification/Check  Dynamic Range  Description=min < u < max  enabled=on  stopWhenAssertionFail=on  export=off  icon=graphic
      settings: SourceProductName=Simulink  SourceProductBaseCode=SL
  Divide1 : Product  Inputs=/*
  Divide2 : Product  Inputs=*/
  Divide5 : Product  Inputs=*/
  Math Function : Math  Operator=reciprocal  SaturateOnIntegerOverflow=on
  Math Function1 : Math  Operator=reciprocal  SaturateOnIntegerOverflow=on
  Math Function2 : Math  Operator=reciprocal  SaturateOnIntegerOverflow=on
  Sum1 : Sum  Inputs=+-
  Sum2 : Sum  Inputs=-+
  Sum5 : Sum  Inputs=+-
  Sum7 : Sum  Inputs=+-
  Thermodynamic property (saturated)1 : thermochemical/Thermodynamic fluid properties/Thermodynamic  property (saturated)  sel=rho(T) vap. (mol/m3)  fluid=fluid  lookup1D_BreakPoint1=fluid.sat.T  lookup1D_Data=fluid.sat.vap.rho_molar
      settings: SourceProductName=@ Thermochemical
  Thermodynamic property (saturated)2 : thermochemical/Thermodynamic fluid properties/Thermodynamic  property (saturated)  sel=rho(T) liq. (mol/m3)  fluid=fluid  lookup1D_BreakPoint1=fluid.sat.T  lookup1D_Data=fluid.sat.liq.rho_molar
      settings: SourceProductName=@ Thermochemical
  dn_gas1 : Constant  Value=1+eps
  dn_gas2 : Constant  Value=1+eps
  dn_gas3 : Constant  Value=-eps
  dn_gas4 : Constant  Value=-eps
  Out1 : Outport
  Out2 : Outport  Port=2
  wires:
  dn_gas1/1 -> Check Dynamic Range1/1
  dn_gas4/1 -> Check Dynamic Range1/2
  dn_gas3/1 -> Check Dynamic Range/2
  dn_gas2/1 -> Check Dynamic Range/1
  N (mol)1/1 -> Divide1/2  "volume (m3)"
  [rho_vap] -> Sum7/2
  [rho] -> Sum7/1
  Divide5/1 -> Out2/1, Check Dynamic Range1/3  "liquid volumetric fraction (0..1)"
  Sum7/1 -> Divide5/1
  [delta_rho] -> Divide5/2
  Divide2/1 -> Out1/1, Check Dynamic Range/3  "vapor quality (0..1)"
  Divide1/1 -> [v], Math Function2/1
  N (mol)/1 -> Divide1/1  "N (mol)"
  Thermodynamic property (saturated)2/1 -> [rho_liq], Math Function/1, Sum5/1
  Thermodynamic property (saturated)1/1 -> [rho_vap], Sum5/2, Math Function1/1
  In1/1 -> Thermodynamic property (saturated)1/1, Thermodynamic property (saturated)2/1  "T (K)"
  Sum1/1 -> Divide2/1
  [v] -> Sum1/1
  [v_liq] -> Sum1/2
  Sum5/1 -> [delta_rho]
  Sum2/1 -> [delta_v]
  Math Function1/1 -> Sum2/2, [v_vap]
  Math Function/1 -> Sum2/1, [v_liq]
  [delta_v] -> Divide2/2
  Math Function2/1 -> [rho]

== system thermochemical/Thermodynamic processes/Isenthalpic throttling outside saturation dome ==
  In3 : Inport
  In4 : Inport  Port=2
  In1 : Inport  Port=3
  Thermodynamic property (non-saturated) : thermochemical/Thermodynamic fluid properties/Thermodynamic  property (non-saturated)  sel=T(h,P)  fluid=fluid  reciprocVar=-1  lookup2D_BreakPoint1=fluid.no_sat.h_P_indep.var_indep.h_molar  lookup2D_BreakPoint2=fluid.no_sat.h_P_indep.var_indep.P  lookup2D_Data=fluid.no_sat.h_P_indep.var_dep.T
      settings: SourceProductName=@ Thermochemical
  Thermodynamic property (non-saturated)1 : thermochemical/Thermodynamic fluid properties/Thermodynamic  property (non-saturated)  sel=h(T,P)  fluid=fluid  reciprocVar=-1  lookup2D_BreakPoint1=fluid.no_sat.T_P_indep.var_indep.T  lookup2D_BreakPoint2=fluid.no_sat.T_P_indep.var_indep.P  lookup2D_Data=fluid.no_sat.T_P_indep.var_dep.h_molar
      settings: SourceProductName=@ Thermochemical
  Out5 : Outport
  Out1 : Outport  Port=2
  wires:
  In1/1 -> Thermodynamic property (non-saturated)/2  "Pout (bar)"
  In4/1 -> Thermodynamic property (non-saturated)1/2  "Pin (bar)"
  In3/1 -> Thermodynamic property (non-saturated)1/1  "Tin (K)"
  Thermodynamic property (non-saturated)/1 -> Out5/1  "Tout (K)"
  Thermodynamic property (non-saturated)1/1 -> Out1/1, Thermodynamic property (non-saturated)/1  "h in = h out (J/mol)"

== system thermochemical/Thermodynamic processes/Mixing chamber (non-saturated) ==
  note: h mix = (dn/dt1*h1+dn/dt2*h2)/(dn/dt1+dn/dt2)
  h1 (J/mol) : Inport
  dN/dt comp (mol/sec) : Inport  Port=2
  h2 (J/mol) : Inport  Port=3
  dn2 (mol/sec) : Inport  Port=4
  dn2 (mol/sec)1 : Inport  Port=5
  Display7 : Display
  Divide : Product  Inputs=*/
  Divide3 : Product  Inputs=**
  Divide5 : Product  Inputs=**
  Sum : Sum
  Sum1 : Sum  Inputs=++|
  Thermodynamic property (non-saturated) : thermochemical/Thermodynamic fluid properties/Thermodynamic  property (non-saturated)  sel=T(h,P)  fluid=fluid  reciprocVar=-1  lookup2D_BreakPoint1=fluid.no_sat.h_P_indep.var_indep.h_molar  lookup2D_BreakPoint2=fluid.no_sat.h_P_indep.var_indep.P  lookup2D_Data=fluid.no_sat.h_P_indep.var_dep.T
      settings: SourceProductName=@ Thermochemical
  Tmix (K) : Outport
  Tmix (K)1 : Outport  Port=2
  wires:
  dn2 (mol/sec)1/1 -> Thermodynamic property (non-saturated)/2  "P (bar)"
  Thermodynamic property (non-saturated)/1 -> Tmix (K)/1  "T mix (K)"
  Sum/1 -> Divide/1
  dN/dt comp (mol/sec)/1 -> Sum1/1, Divide3/2  "dn/dt 1 (mol/sec) ( > 0)"
  h1 (J/mol)/1 -> Divide3/1  "h 1 (J/mol)"
  dn2 (mol/sec)/1 -> Divide5/2, Sum1/2  "dn/dt 2 (mol/sec) ( > 0)"
  h2 (J/mol)/1 -> Divide5/1  "h 2 (J/mol)"
  Divide3/1 -> Sum/1  "J/sec"
  Divide5/1 -> Sum/2  "J/sec"
  Sum1/1 -> Divide/2  "dn/dt1 + dn/dt2"
  Divide/1 -> Thermodynamic property (non-saturated)/1, Tmix (K)1/1, Display7/1  "h mix (J/mol)"

== system thermochemical/Utils/Average computation 1//(T2-T1)*int{x}|t0=T1,tend=T2 (input) ==
  In2 : Inport
  In1 : Inport  Port=2
  Clock : Clock
  Constant : Constant  Value=T1
  Integration window start time1 : Step  Time=T1+0.1  Before=1  After=0  SampleTime=0
  Integrator4 : Integrator  ExternalReset=level hold
  Math Function : Math  Operator=reciprocal  SaturateOnIntegerOverflow=on
  Product : Product
  Sample and Hold : dspsigops/Sample and Hold  trig=Rising edge  initCond=0  latchinput=on
  Sample and Hold1 : dspsigops/Sample and Hold  trig=Rising edge  initCond=0  latchinput=on
  Sum : Sum  Inputs=-+
  Out1 : Outport
  Out2 : Outport  Port=2
  wires:
  Sum/1 -> Math Function/1
  In1/1 -> Sample and Hold1/Trigger, Sample and Hold/Trigger  "T2 latch (rising edge)"
  Sample and Hold/1 -> Sum/2  "T2"
  Clock/1 -> Sample and Hold/1  "simulation time"
  Constant/1 -> Sum/1
  Product/1 -> Out1/1  "AVG{x}"
  Integration window start time1/1 -> Integrator4/2
  In2/1 -> Integrator4/1  "x"
  Sample and Hold1/1 -> Out2/1, Product/1  "int{x}"
  Integrator4/1 -> Sample and Hold1/1
  Math Function/1 -> Product/2  "1/(T2-T1)"

== system thermochemical/Utils/Average computation: 1//(T2-T1)*int{x}|t0=T1,tend=T2 ==
  In2 : Inport
  Gain4 : Gain  Gain=1/(T2-T1)
  Integration window start time1 : Step  Time=T1+0.1  Before=1  After=0  SampleTime=0
  Integration window stop time1 : Step  Time=T2  SampleTime=0
  Integrator4 : Integrator  ExternalReset=level hold
  Sample and Hold : dspsigops/Sample and Hold  trig=Rising edge  initCond=0  latchinput=on
  Sum1 : Sum
  Out1 : Outport
  wires:
  Integration window start time1/1 -> Sum1/1
  Gain4/1 -> Sample and Hold/1
  Integrator4/1 -> Gain4/1
  In2/1 -> Integrator4/1  "x"
  Sum1/1 -> Integrator4/2
  Sample and Hold/1 -> Out1/1  "AVG"
  Integration window stop time1/1 -> Sum1/2, Sample and Hold/Trigger

== system thermochemical/Valves/Upstream//downstream detector ==
  In4 : Inport
  In1 : Inport  Port=2
  In2 : Inport  Port=3
  In3 : Inport  Port=4
  Gain : Gain  Gain=-1
  MinMax : MinMax  Inputs=2
  MinMax1 : MinMax  Function=max  Inputs=2
  Sum : Sum  Inputs=-+
  Switch : Switch  Criteria=u2 > Threshold
  Switch1 : Switch  Criteria=u2 > Threshold
  Out6 : Outport
  Out4 : Outport  Port=2
  Out5 : Outport  Port=3
  Out7 : Outport  Port=4
  wires:
  Gain/1 -> Switch1/2
  In3/1 -> Switch1/3, Switch/3  "T2 (K)"
  In1/1 -> Switch/1, Switch1/1  "T1 (K)"
  MinMax/1 -> Out5/1  "P downstream (bar)"
  In4/1 -> Sum/2, MinMax/1, MinMax1/1  "P1 (bar)"
  Switch/1 -> Out6/1  "T upstream (K)"
  Switch1/1 -> Out7/1  "T downstream (K)"
  MinMax1/1 -> Out4/1  "P upstream (bar)"
  Sum/1 -> Switch/2, Gain/1  "P1 - P2"
  In2/1 -> Sum/1, MinMax/2, MinMax1/2  "P2 (bar)"

== system thermochemical/Valves/Valve, gas, IEC 60534-2-1:2012 (exact) ==
  alpha : Inport
  alpha2 : Inport  Port=2
  alpha3 : Inport  Port=3
  alpha4 : Inport  Port=4
  alpha1 : Inport  Port=5
  1-D Lookup Table : Lookup_n-D  NumberOfTableDimensions=1  BreakpointsForDimension1=apperture_dataPoints  BeginIndexSearchUsingPreviousIndexResult=on  Table=Cv_dataPoints  ExtrapMethod=Clip  InternalRulePriority=Speed  RndMeth=Simplest  InputSameDT=on
  Display5 : Display
  "Flow computation for compressible fluids, IEC 60534-2-1:2012" : Subsystem
  Out2 : Outport
  Out3 : Outport  Port=2
  Out1 : Outport  Port=3
  wires:
  "Flow computation for compressible fluids, IEC 60534-2-1:2012"/1(Out1) -> Out2/1  "W (kg/h)"
  alpha/1 -> 1-D Lookup Table/1  "apperture ([0..1])"
  "Flow computation for compressible fluids, IEC 60534-2-1:2012"/2(Out2) -> Out3/1  "regime"
  1-D Lookup Table/1 -> Out1/1, Display5/1, "Flow computation for compressible fluids, IEC 60534-2-1:2012"/1(In1)  "Cv"
  alpha1/1 -> "Flow computation for compressible fluids, IEC 60534-2-1:2012"/2(In2)  "gamma upstream (1)"
  alpha2/1 -> "Flow computation for compressible fluids, IEC 60534-2-1:2012"/3(In3)  "P upstream (bar)"
  alpha3/1 -> "Flow computation for compressible fluids, IEC 60534-2-1:2012"/4(In4)  "P downstream (bar)"
  alpha4/1 -> "Flow computation for compressible fluids, IEC 60534-2-1:2012"/5(In5)  "rho upstream (kg/m3)"

== system thermochemical/Valves/Valve, gas, IEC 60534-2-1:2012 (modified ideal gas approx.) ==
  alpha : Inport
  alpha2 : Inport  Port=2
  alpha3 : Inport  Port=3
  In1 : Inport  Port=4
  alpha1 : Inport  Port=5
  alpha4 : Inport  Port=6
  In2 : Inport  Port=7
  1-D Lookup Table : Lookup_n-D  NumberOfTableDimensions=1  BreakpointsForDimension1=apperture_dataPoints  BeginIndexSearchUsingPreviousIndexResult=on  Table=Cv_dataPoints  ExtrapMethod=Clip  InternalRulePriority=Speed  RndMeth=Simplest  InputSameDT=on
  Display5 : Display
  "Glow computation for compressible fluids, IEC 60534-2-1:2012 (modified ideal gas assumption)" : Subsystem
  Out2 : Outport
  Out3 : Outport  Port=2
  Out1 : Outport  Port=3
  wires:
  alpha4/1 -> "Glow computation for compressible fluids, IEC 60534-2-1:2012 (modified ideal gas assumption)"/6(In5)  "compressibility factor Z (1)"
  alpha3/1 -> "Glow computation for compressible fluids, IEC 60534-2-1:2012 (modified ideal gas assumption)"/3(In4)  "P downstream (bar)"
  alpha2/1 -> "Glow computation for compressible fluids, IEC 60534-2-1:2012 (modified ideal gas assumption)"/2(In3)  "P upstream (bar)"
  alpha1/1 -> "Glow computation for compressible fluids, IEC 60534-2-1:2012 (modified ideal gas assumption)"/7(gamma upstream (1))  "molecular weight ratio Gg (Mgas/Mair) (1)"
  1-D Lookup Table/1 -> Out1/1, "Glow computation for compressible fluids, IEC 60534-2-1:2012 (modified ideal gas assumption)"/1(In1), Display5/1  "Cv"
  "Glow computation for compressible fluids, IEC 60534-2-1:2012 (modified ideal gas assumption)"/2(Out2) -> Out3/1  "regime"
  alpha/1 -> 1-D Lookup Table/1  "apperture ([0..1])"
  "Glow computation for compressible fluids, IEC 60534-2-1:2012 (modified ideal gas assumption)"/1(Out1) -> Out2/1  "Qs (std m3/h) @ [60°F,1atm]"
  In2/1 -> "Glow computation for compressible fluids, IEC 60534-2-1:2012 (modified ideal gas assumption)"/5(In2)  "gamma upstream (1)"
  In1/1 -> "Glow computation for compressible fluids, IEC 60534-2-1:2012 (modified ideal gas assumption)"/4(In6)  "T upstream (K)"

== system thermochemical/Valves/Valve, gas, Swagelok model ==
  note: Note : dn/dt at any standard condition is equal to dn/dt at real conditions!
  alpha : Inport
  alpha1 : Inport  Port=2
  alpha2 : Inport  Port=3
  alpha3 : Inport  Port=4
  1-D Lookup Table : Lookup_n-D  NumberOfTableDimensions=1  BreakpointsForDimension1=apperture_dataPoints  BeginIndexSearchUsingPreviousIndexResult=on  Table=Cv_dataPoints  ExtrapMethod=Clip  InternalRulePriority=Speed  RndMeth=Simplest  InputSameDT=on
  Display5 : Display
  Gas density (kg/m3) at 'old' standard conditions : Gain  Gain=rho_gas_60F_1atm_kg_m3
  Gas flow computation ('Swagelok' equations) : Subsystem
  Gas molar mass (kg/mol) : Gain  Gain=1/M_gas
  Volume flow rate conversion : thermochemical/Conversions/Volume flow rate conversion  sel=CFH --> m3/sec
      settings: SourceProductName=@ Thermochemical
  Volume flow rate conversion1 : thermochemical/Conversions/Volume flow rate conversion  sel=CFH --> CFM
      settings: SourceProductName=@ Thermochemical
  Out5 : Outport
  Out4 : Outport  Port=2
  Out1 : Outport  Port=3
  Out3 : Outport  Port=4
  Out2 : Outport  Port=5
  wires:
  alpha/1 -> 1-D Lookup Table/1  "apperture ([0..1])"
  Gas flow computation ('Swagelok' equations)/2(Out2) -> Out3/1  "regime"
  1-D Lookup Table/1 -> Display5/1, Out2/1, Gas flow computation ('Swagelok' equations)/1(In1)  "Cv"
  alpha1/1 -> Gas flow computation ('Swagelok' equations)/2(In2)  "T upstream (K)"
  alpha2/1 -> Gas flow computation ('Swagelok' equations)/3(In3)  "P upstream (bar)"
  alpha3/1 -> Gas flow computation ('Swagelok' equations)/4(In4)  "P downstream (bar)"
  Gas flow computation ('Swagelok' equations)/1(Out1) -> Volume flow rate conversion1/1, Volume flow rate conversion/1, Out4/1  "SCFH"
  Gas density (kg/m3) at 'old' standard conditions/1 -> Gas molar mass (kg/mol)/1
  Volume flow rate conversion/1 -> Gas density (kg/m3) at 'old' standard conditions/1
  Gas molar mass (kg/mol)/1 -> Out5/1  "dn/dt (mol/sec)"
  Volume flow rate conversion1/1 -> Out1/1  "SCFM"

== system thermochemical/Valves/Valve, liquid (chocked condition not implemented) ==
  alpha : Inport
  alpha1 : Inport  Port=2
  alpha3 : Inport  Port=3
  In2 : Inport  Port=4
  1-D Lookup Table : Lookup_n-D  NumberOfTableDimensions=1  BreakpointsForDimension1=apperture_dataPoints  BeginIndexSearchUsingPreviousIndexResult=on  Table=Cv_dataPoints  ExtrapMethod=Clip  InternalRulePriority=Speed  RndMeth=Simplest  InputSameDT=on
  Display5 : Display
  Volume flow computation : Subsystem
  Volume flow rate conversion1 : thermochemical/Conversions/Volume flow rate conversion  sel=gpmUS --> m3/h
      settings: SourceProductName=@ Thermochemical
  Volume flow rate conversion2 : thermochemical/Conversions/Volume flow rate conversion  sel=gpmUS --> CFM
      settings: SourceProductName=@ Thermochemical
  Volume flow rate conversion3 : thermochemical/Conversions/Volume flow rate conversion  sel=gpmUS --> L/min
      settings: SourceProductName=@ Thermochemical
  Out4 : Outport
  Out2 : Outport  Port=2
  Out1 : Outport  Port=3
  Out6 : Outport  Port=4
  Out3 : Outport  Port=5
  Out5 : Outport  Port=6
  wires:
  Volume flow computation/2(Out2) -> Out3/1  "regime"
  alpha1/1 -> Volume flow computation/2(In3)  "P upstream (bar)"
  1-D Lookup Table/1 -> Out5/1, Display5/1, Volume flow computation/1(In1)  "Cv"
  Volume flow computation/1(Out1) -> Out4/1, Volume flow rate conversion2/1, Volume flow rate conversion1/1, Volume flow rate conversion3/1  "US gpm"
  Volume flow rate conversion1/1 -> Out1/1  "m3/h"
  alpha/1 -> 1-D Lookup Table/1  "apperture ([0..1])"
  alpha3/1 -> Volume flow computation/3(In4)  "P downstream (bar)"
  Volume flow rate conversion2/1 -> Out2/1  "CFM"
  Volume flow rate conversion3/1 -> Out6/1  "L/min"
  In2/1 -> Volume flow computation/4(In2)  "rho uptream (kg/m3) @ [Tupstream,Pupstream]"

== system thermochemical/Valves/Valve, liquid, IEC 60534-2-1:2012 ==
  alpha : Inport
  In3 : Inport  Port=2
  In4 : Inport  Port=3
  In5 : Inport  Port=4
  P upstream (bar)2 : Inport  Port=5
  P upstream (bar)1 : Inport  Port=6
  1-D Lookup Table : Lookup_n-D  NumberOfTableDimensions=1  BreakpointsForDimension1=apperture_dataPoints  BeginIndexSearchUsingPreviousIndexResult=on  Table=Cv_dataPoints  ExtrapMethod=Clip  InternalRulePriority=Speed  RndMeth=Simplest  InputSameDT=on
  Display5 : Display
  "Flow computation for incompressible fluids, IEC 60534-2-1:2012" : Subsystem
  Volume flow rate conversion1 : thermochemical/Conversions/Volume flow rate conversion  sel=gpmUS --> m3/h
      settings: SourceProductName=@ Thermochemical
  Volume flow rate conversion2 : thermochemical/Conversions/Volume flow rate conversion  sel=gpmUS --> L/min
      settings: SourceProductName=@ Thermochemical
  Volume flow rate conversion3 : thermochemical/Conversions/Volume flow rate conversion  sel=gpmUS --> m3/sec
      settings: SourceProductName=@ Thermochemical
  Out2 : Outport
  Out1 : Outport  Port=2
  Out4 : Outport  Port=3
  Out5 : Outport  Port=4
  Out3 : Outport  Port=5
  Out6 : Outport  Port=6
  wires:
  1-D Lookup Table/1 -> Out6/1, Display5/1, "Flow computation for incompressible fluids, IEC 60534-2-1:2012"/1(In1)  "Cv"
  "Flow computation for incompressible fluids, IEC 60534-2-1:2012"/2(Out2) -> Out3/1  "regime"
  alpha/1 -> 1-D Lookup Table/1  "apperture ([0..1])"
  "Flow computation for incompressible fluids, IEC 60534-2-1:2012"/1(Out1) -> Out2/1, Volume flow rate conversion3/1, Volume flow rate conversion2/1, Volume flow rate conversion1/1  "Q (US gpm)"
  In3/1 -> "Flow computation for incompressible fluids, IEC 60534-2-1:2012"/2(In3)  "P upstream (bar)"
  In4/1 -> "Flow computation for incompressible fluids, IEC 60534-2-1:2012"/3(In4)  "P downstream (bar)"
  P upstream (bar)2/1 -> "Flow computation for incompressible fluids, IEC 60534-2-1:2012"/4(P upstream (bar)2)  "Pv: absolute vapor pressure  of liquid at T upstream (bar)"
  In5/1 -> "Flow computation for incompressible fluids, IEC 60534-2-1:2012"/6(In5)  "rho upstream (kg/m3)"
  P upstream (bar)1/1 -> "Flow computation for incompressible fluids, IEC 60534-2-1:2012"/5(P upstream (bar)1)  "Pc: absolute thermodynamic  critical pressure (bar)"
  Volume flow rate conversion3/1 -> Out4/1  "Q (m3/sec)"
  Volume flow rate conversion2/1 -> Out5/1  "Q (L/min)"
  Volume flow rate conversion1/1 -> Out1/1  "Q (m3/h)"

== system thermochemical/Walls/Fin efficiency ==
  h_outer (W/m2/K) : Inport
  Constant5 : Constant
  Constant8 : Constant
  Divide : Product  Inputs=*/
  Divide1 : Product  Inputs=*//
  Divide3 : Product  Inputs=*/
  Divide4 : Product  Inputs=***
  Gain : Gain  Gain=1e-3
  Gain1 : Gain  Gain=2
  Gain2 : Gain  Gain=0.35
  Gain3 : Gain  Gain=1e-3
  Gain4 : Gain  Gain=1e-3
  Gain5 : Gain  Gain=0.5
  Height : Constant  Value=height_fin_mm
  Math Function1 : Math  Operator=log  SaturateOnIntegerOverflow=on
  Outer diameter : Constant  Value=D_mm
  Square root : Subsystem
  Sum : Sum  Inputs=|++
  Sum2 : Sum  Inputs=|++
  Thermal conductivity : Constant  Value=lambda
  Thickness : Constant  Value=thickness_fin_mm
  Trigonometric Function : Trigonometry  Operator=tanh
  eta_fin : Outport
  wires:
  Divide/1 -> eta_fin/1  "eta_fin"
  Math Function1/1 -> Gain2/1
  Gain/1 -> Divide1/2  "t_m"
  Height/1 -> Gain3/1
  Sum2/1 -> Divide4/3  "phi"
  Constant8/1 -> Sum2/2
  Gain2/1 -> Sum2/1
  Gain4/1 -> Divide3/2  "r_m"
  Thermal conductivity/1 -> Divide1/3
  Gain1/1 -> Divide1/1
  Trigonometric Function/1 -> Divide/1
  Outer diameter/1 -> Gain5/1
  Divide4/1 -> Trigonometric Function/1, Divide/2  "arg"
  Constant5/1 -> Sum/2
  Gain3/1 -> Divide4/2, Divide3/1  "L_m"
  Sum/1 -> Math Function1/1
  Divide3/1 -> Sum/1
  h_outer (W/m2/K)/1 -> Gain1/1  "h_outer (W/m²/K)"
  Thickness/1 -> Gain/1
  Gain5/1 -> Gain4/1  "r_mm"
  Divide1/1 -> Square root/1(In1)
  Square root/1(m) -> Divide4/1  "m"
